simulink model "GenericPhaseSteer"  (R2019b)
settings: configuration reference "cset" (kept outside this file)
libraries: simulink_extras x2
settings Model: OrderedModelArguments=off  Creator=tom  LastModifiedBy=tom
settings ConfigSetRef: SourceName=cset  SourceLocation=Base Workspace

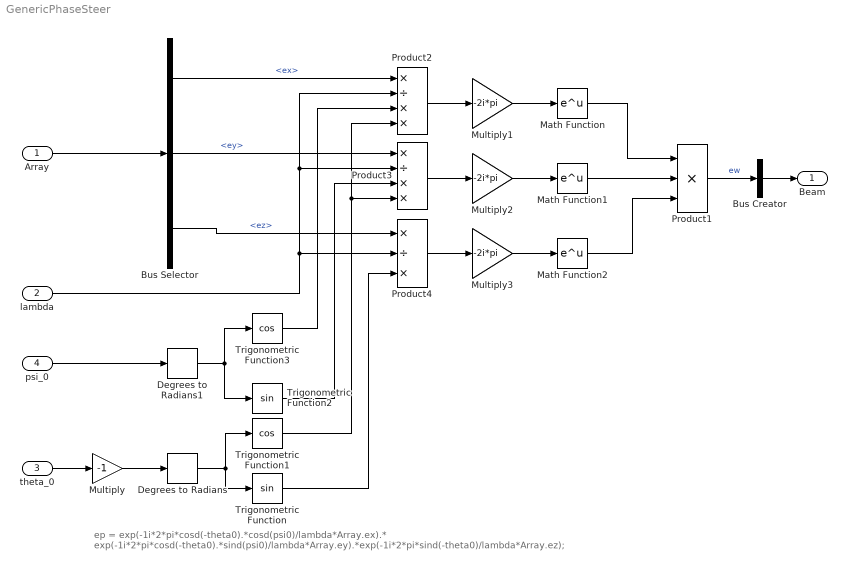
== system GenericPhaseSteer ==
  note: ep = exp(-1i*2*pi*cosd(-theta0).*cosd(psi0)/lambda*Array.ex).* exp(-1i*2*pi*cosd(-theta0).*sind(psi0)/lambda*Array.ey).*exp(-1i*2*pi*sind(-theta0)/lambda*Array.ez);
  Array : Inport  OutDataTypeStr=Bus: SonarWorkbenchArrayObj  PortDimensions=1
  lambda : Inport  Port=2  OutDataTypeStr=double  Unit=1/m  PortDimensions=1
  theta_0 : Inport  Port=3  OutDataTypeStr=double  Unit=deg  PortDimensions=1
  psi_0 : Inport  Port=4  OutDataTypeStr=double  Unit=deg  PortDimensions=1
  Bus Creator : BusCreator  Inputs=1  OutDataTypeStr=Bus: SonarWorkbenchBeamObj
  Bus Selector : BusSelector  OutputSignals=ex,ey,ez
  Degrees to Radians : simulink_extras/Transformations/Degrees to Radians
  Degrees to Radians1 : simulink_extras/Transformations/Degrees to Radians
  Math Function : Math  SignedPower=off  SaturateOnIntegerOverflow=on
  Math Function1 : Math  SignedPower=off  SaturateOnIntegerOverflow=on
  Math Function2 : Math  SignedPower=off  SaturateOnIntegerOverflow=on
  Multiply : Gain  Gain=-1
  Multiply1 : Gain  Gain=-2i*pi
  Multiply2 : Gain  Gain=-2i*pi
  Multiply3 : Gain  Gain=-2i*pi
  Product1 : Product  Inputs=3
  Product2 : Product  Inputs=*/**
  Product3 : Product  Inputs=*/**
  Product4 : Product  Inputs=*/*
  Trigonometric Function : Trigonometry
  Trigonometric Function1 : Trigonometry  Operator=cos
  Trigonometric Function2 : Trigonometry
  Trigonometric Function3 : Trigonometry  Operator=cos
  Beam : Outport  OutDataTypeStr=Bus: SonarWorkbenchBeamObj  PortDimensions=1
  wires:
  Degrees to Radians/1 -> Trigonometric Function1/1, Trigonometric Function/1
  psi_0/1 -> Degrees to Radians1/1
  Degrees to Radians1/1 -> Trigonometric Function3/1, Trigonometric Function2/1
  theta_0/1 -> Multiply/1
  Array/1 -> Bus Selector/1
  Multiply/1 -> Degrees to Radians/1
  Bus Selector/1 -> Product2/1  "<ex>"
  lambda/1 -> Product4/2, Product3/2, Product2/2
  Trigonometric Function1/1 -> Product2/4, Product3/4
  Trigonometric Function3/1 -> Product2/3
  Bus Selector/2 -> Product3/1  "<ey>"
  Trigonometric Function2/1 -> Product3/3
  Bus Selector/3 -> Product4/1  "<ez>"
  Trigonometric Function/1 -> Product4/3
  Product2/1 -> Multiply1/1
  Product3/1 -> Multiply2/1
  Product4/1 -> Multiply3/1
  Multiply1/1 -> Math Function/1
  Multiply2/1 -> Math Function1/1
  Multiply3/1 -> Math Function2/1
  Math Function/1 -> Product1/1
  Math Function1/1 -> Product1/2
  Math Function2/1 -> Product1/3
  Product1/1 -> Bus Creator/1  "ew"
  Bus Creator/1 -> Beam/1
